simulink model "DC_Motor_PI"  (R2023a)
settings: Solver=ode45  StartTime=0.0  StopTime=10  RelTol=1e-3  EnableMultiTasking=on
libraries: simulink_need_slupdate x1
settings Model: Creator=VICTOR  LastModifiedBy=dhana
settings SolverCC: AlgebraicLoopSolver=TrustRegion
settings DataIOCC: LimitDataPoints=on  SaveFormat=Array  SignalLoggingSaveFormat=ModelDataLogs  ReturnWorkspaceOutputs=off
settings OptimizationCC: ExpressionDepthLimit=2147483647  InitFltsAndDblsToZero=on  LifeSpan=inf
settings DebuggingCC: UnderspecifiedInitializationDetection=Classic  MergeDetectMultiDrivingBlocksExec=none  SolverPrmCheckMsg=warning  FcnCallInpInsideContextMsg=warning  UnconnectedInputMsg=warning  UnconnectedOutputMsg=warning  UnconnectedLineMsg=warning  StateNameClashWarn=warning  SFUnexpectedBacktrackingDiag=warning  SFNoUnconditionalDefaultTransitionDiag=warning  SFExecutionAtInitializationDiag=none  ArithmeticOperatorsInVariantConditions=warning
settings HardwareCC: ProdBitPerPointer=32  ProdBitPerSizeT=32  ProdBitPerPtrDiffT=32  ProdLargestAtomicFloat=None  ProdIntDivRoundTo=Undefined  ProdEndianess=Unspecified  ProdWordSize=32  ProdHWDeviceType=32-bit Generic
settings ModelReferenceCC: PropagateSignalLabelsOutOfModel=off
settings SFSimCC: SimUseLocalCustomCode=off  CustomCodeUndefinedFunction=UseInterfaceOnly
settings RTWCC: RTWUseLocalCustomCode=off
settings CodeAppCC: StateflowObjectComments=on
settings GRTTargetCC: TargetLangStandard=C89/C90 (ANSI)  CombineOutputUpdateFcns=off  GRTInterface=on
settings ConfigComp: CovMetricSettings=dw  CovSaveCumulativeToWorkspaceVar=on  CovSaveSingleToWorkspaceVar=on  CovExternalEMLEnable=off  CovSFcnEnable=off
settings SimscapeCC: SimscapeNormalizeSystem=off
settings ConfigurationSet: Description=SimMechanics 2G

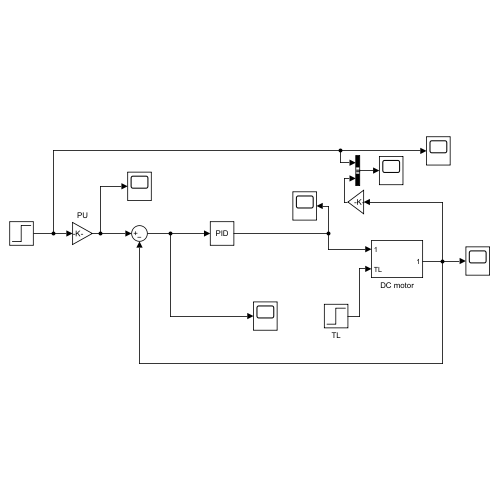
[thumbnail: Simulink's stored preview of the top-level diagram]
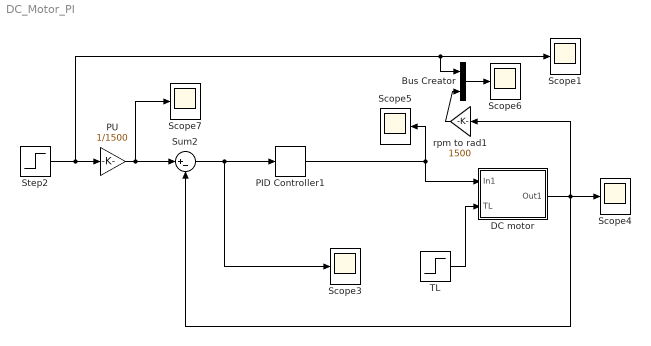
== system DC_Motor_PI ==
  Bus Creator : BusCreator  Inputs=2
  DC motor : Subsystem  mask{Ra=1, La=0.5, J=0.01, D=0.1}
      mask prompts: Ra "Armature Resistance (Ra)"; La "Armature Inductance (La)"; J "Inertia (J)"; D "Damping (B)"
  PID Controller1 : simulink_need_slupdate/PID Controller  P=2  I=10  D=0
  PU : Gain  Gain=1/1500
  Scope{1,3..7} (6 alike) : Scope
  Step2 : Step  Time=5  Before=800  After=1450  SampleTime=0.0001
  Sum2 : Sum  Inputs=|+-
  TL : Step  Time=7  Before=0.0001  After=0.002  SampleTime=0
  rpm to rad1 : Gain  Gain=1500
  wires:
  Step2/1 -> Bus Creator/1, Scope1/1, PU/1
  Sum2/1 -> Scope3/1, PID Controller1/1
  DC motor/1(Out1) -> Sum2/2, rpm to rad1/1, Scope4/1
  PID Controller1/1 -> DC motor/1(In1), Scope5/1
  Bus Creator/1 -> Scope6/1
  rpm to rad1/1 -> Bus Creator/2
  PU/1 -> Sum2/1, Scope7/1
  TL/1 -> DC motor/2(TL)

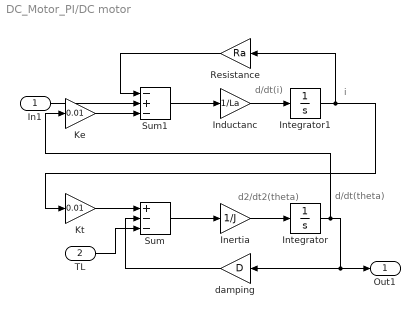
== system DC_Motor_PI/DC motor ==
  note: d/dt(i)
  note: i
  note: d/dt(theta)
  note: d2/dt2(theta)
  In1 : Inport
  TL : Inport  Port=2
  Inductanc : Gain  Gain=1/La  SaturateOnIntegerOverflow=on  OutDataTypeStr=Inherit: Same as input  ParamDataTypeStr=Inherit: Same as input
  Inertia : Gain  Gain=1/J  SaturateOnIntegerOverflow=on  OutDataTypeStr=Inherit: Same as input  ParamDataTypeStr=Inherit: Same as input
  Integrator : Integrator
  Integrator1 : Integrator
  Ke : Gain  Gain=0.01  SaturateOnIntegerOverflow=on  OutDataTypeStr=Inherit: Same as input  ParamDataTypeStr=Inherit: Same as input
  Kt : Gain  Gain=0.01  SaturateOnIntegerOverflow=on  OutDataTypeStr=Inherit: Same as input  ParamDataTypeStr=Inherit: Same as input
  Resistance : Gain  Gain=Ra  SaturateOnIntegerOverflow=on  OutDataTypeStr=Inherit: Same as input  ParamDataTypeStr=Inherit: Same as input
  Sum : Sum  Inputs=+--  InputSameDT=on  SaturateOnIntegerOverflow=on  OutDataTypeStr=Inherit: Same as first input
  Sum1 : Sum  Inputs=-+-  InputSameDT=on  SaturateOnIntegerOverflow=on  OutDataTypeStr=Inherit: Same as first input
  damping : Gain  Gain=D  SaturateOnIntegerOverflow=on  OutDataTypeStr=Inherit: Same as input  ParamDataTypeStr=Inherit: Same as input
  Out1 : Outport
  wires:
  Integrator1/1 -> Resistance/1, Kt/1
  Integrator/1 -> Ke/1, damping/1, Out1/1
  Ke/1 -> Sum1/3
  Resistance/1 -> Sum1/1
  Kt/1 -> Sum/1
  damping/1 -> Sum/2
  Sum1/1 -> Inductanc/1
  Sum/1 -> Inertia/1
  Inertia/1 -> Integrator/1
  Inductanc/1 -> Integrator1/1
  In1/1 -> Sum1/2
  TL/1 -> Sum/3
